simulink model "plant_block_swing_catch"  (R2013a)
settings: Solver=ode1  StartTime=0.0  StopTime=420  RelTol=1e-3
undefined symbols (not defined in the file or in its folder): magnitude
libraries: simulink x11
settings Model: SimulationMode=external  ExtModeTrigDuration=50000  Creator=Dro  LastModifiedBy=s4358046
settings DataIOCC: LimitDataPoints=off  SignalLoggingSaveFormat=ModelDataLogs  SignalLoggingName=sigsOut
settings OptimizationCC: ExpressionDepthLimit=2147483647  InitFltsAndDblsToZero=on
settings DebuggingCC: SaveWithParameterizedLinksMsg=none  SignalResolutionControl=TryResolveAllWithWarning  SolverPrmCheckMsg=none  MultiTaskDSMMsg=warning  MultiTaskCondExecSysMsg=none  FcnCallInpInsideContextMsg=UseLocalSettings  StrictBusMsg=None
settings RTWCC: SystemTargetFile=rtwin.tlc  TemplateMakefile=rtwin.tmf  Description=Real-Time Windows Target  ProcessScript=rtwin_make_rtw_hook  IncludeERTFirstTime=on
settings RTWinTargetCC: TargetFcnLib=ansi_tfl_tmw.mat  TargetLibSuffix=_rtwin.lib  TargetPreCompLibLocation=C:\Program Files\MATLAB\R2013a\toolbox\rtw\targets\rtwin\lib\win64  CodeReplacementLibrary=ANSI_C  ModelReferenceCompliant=off  CompOptLevelCompliant=off  RTWinDir=C:/PROGRA~1/MATLAB/R2013a/toolbox/rtw/targets/rtwin  TargetArch=win64

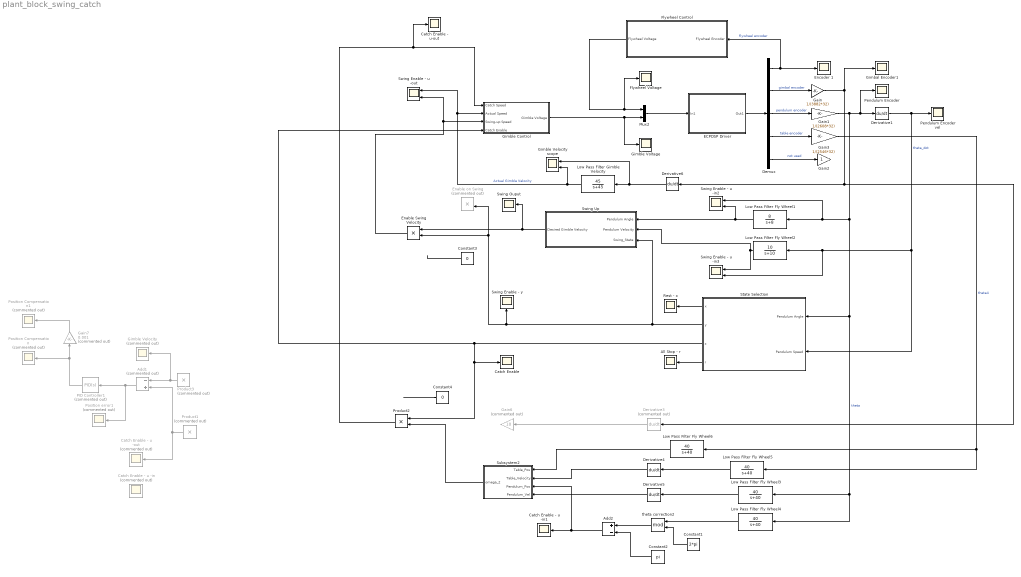
== system plant_block_swing_catch ==
  Add1 : Sum  Commented=on  Inputs=-+
  Add2 : Sum  Inputs=+-
  All Stop - r : Scope
      settings: YMin=-10  YMax=10  SaveName=ScopeData33
  Catch Enable : Scope
      settings: YMin=-10  YMax=10  SaveName=ScopeData12
  Catch Enable - u -in : Scope  Commented=on
      settings: YMin=-10  YMax=10  SaveName=ScopeData2
  Catch Enable - u -in1 : Scope
      settings: YMin=-10  YMax=10  SaveName=ScopeData26
  Catch Enable - u -out : Scope  Commented=on
      settings: YMin=-10  YMax=10  SaveName=ScopeData8
  Catch Enable - u-out : Scope
      settings: YMin=-10  YMax=10  SaveName=ScopeData20
  Constant1 : Constant  Value=2*pi
  Constant2 : Constant  Value=pi
  Constant3 : Constant  Value=0
  Constant4 : Constant  Value=0
  Demux : Demux  Outputs=5
  Derivative{1,4..6} (4 alike) : Derivative
  Derivative3 : Derivative  Commented=on
  ECPDSP Driver : Subsystem  mask{BaseAddr='0xC000', STime=0.008, TimeOutPer=500, HWAccess=on}
      mask prompts: BaseAddr "Base I/O Address"; STime "Sample Time (Sec)"; TimeOutPer "Timeout Period (500 ~ 2000)"; HWAccess "Hardware Access"
      mask Display: color('black');disp('ECPDSP Driver\n upto\n 4 Encs(ADC Channels)\n and 2 Dacs')
  Enable Swing Velocity : Product
  Enable on Swing : Product  Commented=on
  Encoder 1 : Scope
      settings: YMin=1.5e+06  YMax=8.5e+06  SaveName=ScopeData3
  Flywheel Control : Subsystem
  Flywheel Voltage : Scope
      settings: YMin=30400  YMax=33600  SaveName=ScopeData6
  Gain : Gain  Gain=1/(3882*32)
  Gain1 : Gain  Gain=1/(2608*32)
  Gain2 : Gain
  Gain3 : Gain  Gain=1/(2546*32)
  Gain6 : Gain  Commented=on  Gain=10
  Gain7 : Gain  Commented=on  Gain=0.001
  Gimbal Encoder1 : Scope
      settings: YMin=-0.25  YMax=3.25  SaveName=ScopeData9
  Gimble Control : Subsystem
  Gimble Velocity : Scope  Commented=on
      settings: YMin=-10  YMax=10  SaveName=ScopeData10
  Gimble Velocity scope : Scope  NumInputPorts=2
      settings: YMin=-10~-5  YMax=10~5  SaveName=ScopeData32
  Gimble Voltage : Scope
      settings: TimeRange=4.21022074346109  YMin=-27910.40741056809  YMax=13910.18606424908  SaveName=ScopeData23
  Low Pass Filter Fly Wheel1 : TransferFcn  Numerator=[8]  Denominator=[1 8]
  Low Pass Filter Fly Wheel2 : TransferFcn  Numerator=[10]  Denominator=[1 10]
  Low Pass Filter Fly Wheel{3..6} (4 alike) : TransferFcn  Numerator=[40]  Denominator=[1 40]
  Low Pass Filter Gimble Velocity : TransferFcn  Numerator=[45]  Denominator=[1 45]
  Mux2 : Mux  Inputs=2
  PID Controller1 : simulink/Continuous/PID Controller  Commented=on  Controller=PID  TimeDomain=Continuous-time  SampleTime=1  IntegratorMethod=Forward Euler  FilterMethod=Forward Euler  Form=Parallel  P=200  I=50  D=0  N=100  InitialConditionSource=internal  InitialConditionForIntegrator=0  InitialConditionForFilter=0  ExternalReset=none  LimitOutput=off  UpperSaturationLimit=inf  LowerSaturationLimit=-inf  LinearizeAsGain=on  AntiWindupMode=none  Kb=1  TrackingMode=off  Kt=1  PParamMin=[]  PParamMax=[]  IParamMin=[]  IParamMax=[]  DParamMin=[]  DParamMax=[]  NParamMin=[]  NParamMax=[]  KbParamMin=[]  KbParamMax=[]  KtParamMin=[]  KtParamMax=[]  POutMin=[]  POutMax=[]  IOutMin=[]  IOutMax=[]  DOutMin=[]  DOutMax=[]  NOutMin=[]  NOutMax=[]  KbOutMin=[]  KbOutMax=[]  KtOutMin=[]  KtOutMax=[]  IntegratorOutMin=[]  IntegratorOutMax=[]  FilterOutMin=[]  FilterOutMax=[]  SumOutMin=[]  SumOutMax=[]  SumI1OutMin=[]  SumI1OutMax=[]  SumI2OutMin=[]  SumI2OutMax=[]  SumI3OutMin=[]  SumI3OutMax=[]  SumDOutMin=[]  SumDOutMax=[]  SaturationOutMin=[]  SaturationOutMax=[]  IntegratorContinuousStateAttributes=''  IntegratorStateMustResolveToSignalObject=off  IntegratorRTWStateStorageClass=Auto  FilterContinuousStateAttributes=''  FilterStateMustResolveToSignalObject=off  FilterRTWStateStorageClass=Auto
  Pendulum Encoder : Scope
      settings: YMin=-3.175  YMax=-3.1  SaveName=ScopeData5
  Pendulum Encoder vel : Scope
      settings: YMin=-0.25  YMax=3.25  SaveName=ScopeData19
  Position Compensation : Scope  Commented=on
      settings: YMin=-10  YMax=10  SaveName=ScopeData11
  Position Compensation1 : Scope  Commented=on
      settings: YMin=-10  YMax=10  SaveName=ScopeData13
  Position error1 : Scope  Commented=on
      settings: YMin=-10  YMax=10  SaveName=ScopeData14
  Product1 : Product  Commented=on
  Product2 : Product
  Product3 : Product  Commented=on
  Rest - x : Scope
      settings: YMin=-10  YMax=10  SaveName=ScopeData15
  State Selection : Subsystem
  Subsystem2 : Subsystem
  Swing Enable - u -in2 : Scope  NumInputPorts=2
      settings: YMin=-10~-5  YMax=10~5  SaveName=ScopeData30
  Swing Enable - u -in3 : Scope  NumInputPorts=2
      settings: YMin=-10~-5  YMax=10~5  SaveName=ScopeData31
  Swing Enable - u -out : Scope  NumInputPorts=2
      settings: YMin=-10~-5  YMax=10~5  SaveName=ScopeData18
  Swing Enable - y : Scope
      settings: YMin=-10  YMax=10  SaveName=ScopeData16
  Swing Ouput : Scope
      settings: YMin=-10  YMax=10  SaveName=ScopeData17
  Swing Up : Subsystem
  theta correction2 : Math  Operator=mod  SaturateOnIntegerOverflow=on
  wires:
  ECPDSP Driver/1(Out1) -> Demux/1
  Demux/1 -> Encoder 1/1, Flywheel Control/1(Flywheel Encoder)  "flywheel encoder"
  Demux/2 -> Gain/1  "gimbal encoder"
  Demux/3 -> Gain1/1  "pendulum encoder"
  Demux/4 -> Gain3/1  "table encoder"
  Demux/5 -> Gain2/1  "not used"
  Derivative1/1 -> State Selection/2(Pendulum Speed), Swing Enable - u -in3/2, Low Pass Filter Fly Wheel2/1, Pendulum Encoder vel/1  "theta_dot"
  Gain1/1 -> Low Pass Filter Fly Wheel3/1, Low Pass Filter Fly Wheel4/1, State Selection/1(Pendulum Angle), Swing Enable - u -in2/1, Low Pass Filter Fly Wheel1/1, Pendulum Encoder/1, Derivative1/1  "theta"
  Swing Up/1(Desired Gimble Velocity) -> Swing Ouput/1, Enable Swing Velocity/1
  Subsystem2/1(omega_2) -> Product2/2
  Derivative3/1 -> Gain6/1
  theta correction2/1 -> Add2/1
  Add2/1 -> Subsystem2/3(Pendulum_Pos), Catch Enable - u -in1/1
  Mux2/1 -> ECPDSP Driver/1(In1)
  Derivative4/1 -> Subsystem2/2(Table_Velocity)
  Constant1/1 -> theta correction2/2
  Constant2/1 -> Add2/2
  Derivative6/1 -> Low Pass Filter Gimble Velocity/1, Gimble Velocity scope/1
  Low Pass Filter Fly Wheel2/1 -> Swing Up/2(Pendulum Velocity), Swing Enable - u -in3/1
  Low Pass Filter Gimble Velocity/1 -> Gimble Velocity scope/2, Swing Enable - u -out/1, Gimble Control/2(Actual Speed)  "Actual Gimble Velocity"
  Low Pass Filter Fly Wheel1/1 -> Swing Enable - u -in2/2, Swing Up/1(Pendulum Angle)
  Enable Swing Velocity/1 -> Swing Enable - u -out/2, Gimble Control/3(Swing-up Speed)
  Flywheel Control/1(Flywheel Voltage) -> Flywheel Voltage/1, Mux2/1
  Gimble Control/1(Gimble Voltage) -> Mux2/2, Gimble Voltage/1
  State Selection/2(y) -> Enable Swing Velocity/2, Enable on Swing/2, Swing Enable - y/1, Swing Up/3(Swing_State)
  State Selection/1(x) -> Rest - x/1
  State Selection/4(r) -> All Stop - r/1
  Gain3/1 -> Low Pass Filter Fly Wheel5/1, Low Pass Filter Fly Wheel6/1  "theta4"
  Constant3/1 -> ?
  Gain/1 -> Derivative3/1, Derivative6/1, Gimbal Encoder1/1
  ? -> Catch Enable - u -in/1
  ? -> Product1/2
  Add1/1 -> Position error1/1, PID Controller1/1
  Product3/1 -> Gimble Velocity/1, Add1/1
  Product1/1 -> Catch Enable - u -out/1, Add1/2
  ? -> Product3/1
  PID Controller1/1 -> Position Compensation/1, Gain7/1
  Gain7/1 -> Position Compensation1/1
  ? -> Product3/2
  ? -> Product1/1
  Product2/1 -> Catch Enable - u-out/1, Gimble Control/1(Catch Speed)
  Constant4/1 -> ?
  State Selection/3(z) -> Gimble Control/4(Catch Enable), Product2/1, Catch Enable/1
  Low Pass Filter Fly Wheel4/1 -> theta correction2/1
  Derivative5/1 -> Subsystem2/4(Pendulum_Vel)
  Low Pass Filter Fly Wheel3/1 -> Derivative5/1
  Low Pass Filter Fly Wheel5/1 -> Derivative4/1
  Low Pass Filter Fly Wheel6/1 -> Subsystem2/1(Table_Pos)

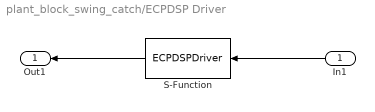
== system plant_block_swing_catch/ECPDSP Driver ==
  In1 : Inport
  S-Function : S-Function  FunctionName=ECPDSPDriver  Parameters=BaseAddr,STime,TimeOutPer,HWAccess  EnableBusSupport=off
  Out1 : Outport
  wires:
  In1/1 -> S-Function/1
  S-Function/1 -> Out1/1

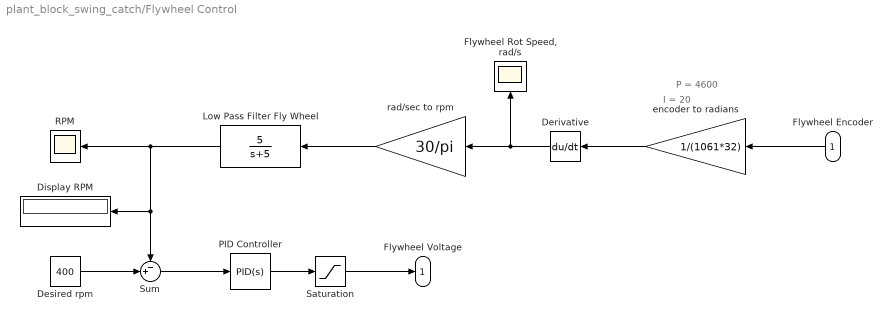
== system plant_block_swing_catch/Flywheel Control ==
  note: I = 20
  note: P = 4600
  Flywheel Encoder : Inport
  Derivative : Derivative
  Desired rpm : Constant  Value=400
  Display RPM : Display
  "Flywheel Rot Speed, rad/s" : Scope
      settings: SaveName=ScopeData4
  Low Pass Filter Fly Wheel : TransferFcn  Numerator=[5]  Denominator=[1 5]
  PID Controller : simulink/Continuous/PID Controller  Controller=PID  TimeDomain=Continuous-time  SampleTime=1  IntegratorMethod=Forward Euler  FilterMethod=Forward Euler  Form=Parallel  P=4600  I=20  D=0  N=100  InitialConditionSource=internal  InitialConditionForIntegrator=0  InitialConditionForFilter=0  ExternalReset=none  LimitOutput=off  UpperSaturationLimit=inf  LowerSaturationLimit=-inf  LinearizeAsGain=on  AntiWindupMode=none  Kb=1  TrackingMode=off  Kt=1  PParamMin=[]  PParamMax=[]  IParamMin=[]  IParamMax=[]  DParamMin=[]  DParamMax=[]  NParamMin=[]  NParamMax=[]  KbParamMin=[]  KbParamMax=[]  KtParamMin=[]  KtParamMax=[]  POutMin=[]  POutMax=[]  IOutMin=[]  IOutMax=[]  DOutMin=[]  DOutMax=[]  NOutMin=[]  NOutMax=[]  KbOutMin=[]  KbOutMax=[]  KtOutMin=[]  KtOutMax=[]  IntegratorOutMin=[]  IntegratorOutMax=[]  FilterOutMin=[]  FilterOutMax=[]  SumOutMin=[]  SumOutMax=[]  SumI1OutMin=[]  SumI1OutMax=[]  SumI2OutMin=[]  SumI2OutMax=[]  SumI3OutMin=[]  SumI3OutMax=[]  SumDOutMin=[]  SumDOutMax=[]  SaturationOutMin=[]  SaturationOutMax=[]  IntegratorContinuousStateAttributes=''  IntegratorStateMustResolveToSignalObject=off  IntegratorRTWStateStorageClass=Auto  FilterContinuousStateAttributes=''  FilterStateMustResolveToSignalObject=off  FilterRTWStateStorageClass=Auto
  RPM : Scope
      settings: YMin=401.6  YMax=403.9
  Saturation : Saturate  UpperLimit=32000  LowerLimit=-32000
  Sum : Sum  Inputs=-+|
  encoder to radians : Gain  Gain=1/(1061*32)
  rad/sec to rpm : Gain  Gain=30/pi
  Flywheel Voltage : Outport
  wires:
  Saturation/1 -> Flywheel Voltage/1
  Sum/1 -> PID Controller/1
  Desired rpm/1 -> Sum/2
  rad/sec to rpm/1 -> Low Pass Filter Fly Wheel/1
  Derivative/1 -> "Flywheel Rot Speed, rad/s"/1, rad/sec to rpm/1
  encoder to radians/1 -> Derivative/1
  Low Pass Filter Fly Wheel/1 -> Sum/1, Display RPM/1, RPM/1
  PID Controller/1 -> Saturation/1
  Flywheel Encoder/1 -> encoder to radians/1

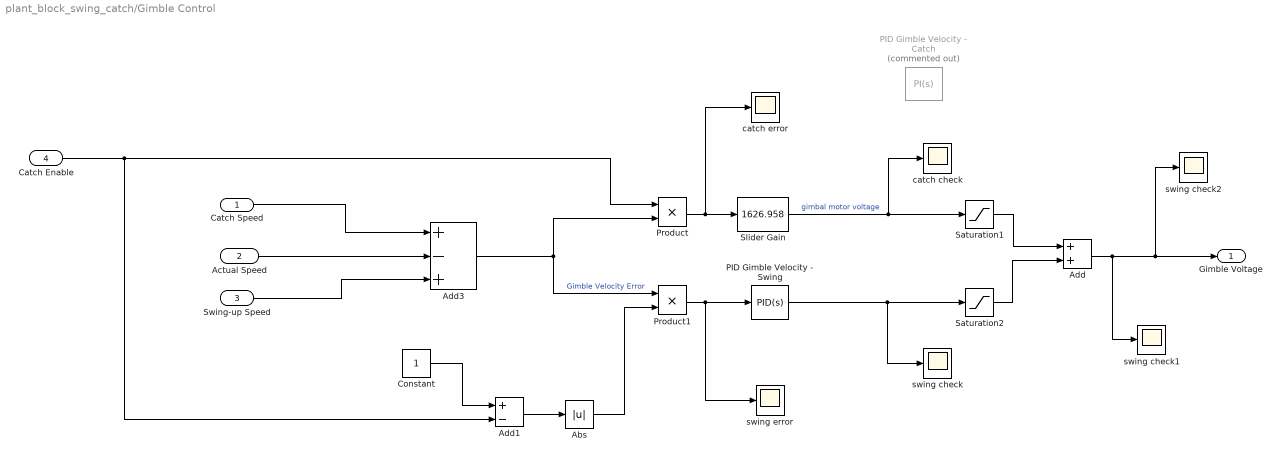
== system plant_block_swing_catch/Gimble Control ==
  Catch Speed : Inport
  Actual Speed : Inport  Port=2
  Swing-up Speed : Inport  Port=3
  Catch Enable : Inport  Port=4
  Abs : Abs
  Add : Sum
  Add1 : Sum  Inputs=+-
  Add3 : Sum  Inputs=+-+
  Constant : Constant
  PID Gimble Velocity - Catch : simulink/Continuous/PID Controller  Commented=on  Controller=PI  TimeDomain=Continuous-time  SampleTime=1  IntegratorMethod=Forward Euler  FilterMethod=Forward Euler  Form=Parallel  P=1000  I=0  D=0  N=100  InitialConditionSource=internal  InitialConditionForIntegrator=0  InitialConditionForFilter=0  ExternalReset=none  LimitOutput=off  UpperSaturationLimit=inf  LowerSaturationLimit=-inf  LinearizeAsGain=on  AntiWindupMode=none  Kb=1  TrackingMode=off  Kt=1  PParamMin=[]  PParamMax=[]  IParamMin=[]  IParamMax=[]  DParamMin=[]  DParamMax=[]  NParamMin=[]  NParamMax=[]  KbParamMin=[]  KbParamMax=[]  KtParamMin=[]  KtParamMax=[]  POutMin=[]  POutMax=[]  IOutMin=[]  IOutMax=[]  DOutMin=[]  DOutMax=[]  NOutMin=[]  NOutMax=[]  KbOutMin=[]  KbOutMax=[]  KtOutMin=[]  KtOutMax=[]  IntegratorOutMin=[]  IntegratorOutMax=[]  FilterOutMin=[]  FilterOutMax=[]  SumOutMin=[]  SumOutMax=[]  SumI1OutMin=[]  SumI1OutMax=[]  SumI2OutMin=[]  SumI2OutMax=[]  SumI3OutMin=[]  SumI3OutMax=[]  SumDOutMin=[]  SumDOutMax=[]  SaturationOutMin=[]  SaturationOutMax=[]  IntegratorContinuousStateAttributes=''  IntegratorStateMustResolveToSignalObject=off  IntegratorRTWStateStorageClass=Auto  FilterContinuousStateAttributes=''  FilterStateMustResolveToSignalObject=off  FilterRTWStateStorageClass=Auto
  PID Gimble Velocity - Swing : simulink/Continuous/PID Controller  Controller=PID  TimeDomain=Continuous-time  SampleTime=1  IntegratorMethod=Forward Euler  FilterMethod=Forward Euler  Form=Parallel  P=12000  I=2500  D=0  N=100  InitialConditionSource=internal  InitialConditionForIntegrator=0  InitialConditionForFilter=0  ExternalReset=none  LimitOutput=off  UpperSaturationLimit=inf  LowerSaturationLimit=-inf  LinearizeAsGain=on  AntiWindupMode=none  Kb=1  TrackingMode=off  Kt=1  PParamMin=[]  PParamMax=[]  IParamMin=[]  IParamMax=[]  DParamMin=[]  DParamMax=[]  NParamMin=[]  NParamMax=[]  KbParamMin=[]  KbParamMax=[]  KtParamMin=[]  KtParamMax=[]  POutMin=[]  POutMax=[]  IOutMin=[]  IOutMax=[]  DOutMin=[]  DOutMax=[]  NOutMin=[]  NOutMax=[]  KbOutMin=[]  KbOutMax=[]  KtOutMin=[]  KtOutMax=[]  IntegratorOutMin=[]  IntegratorOutMax=[]  FilterOutMin=[]  FilterOutMax=[]  SumOutMin=[]  SumOutMax=[]  SumI1OutMin=[]  SumI1OutMax=[]  SumI2OutMin=[]  SumI2OutMax=[]  SumI3OutMin=[]  SumI3OutMax=[]  SumDOutMin=[]  SumDOutMax=[]  SaturationOutMin=[]  SaturationOutMax=[]  IntegratorContinuousStateAttributes=''  IntegratorStateMustResolveToSignalObject=off  IntegratorRTWStateStorageClass=Auto  FilterContinuousStateAttributes=''  FilterStateMustResolveToSignalObject=off  FilterRTWStateStorageClass=Auto
  Product : Product
  Product1 : Product
  Saturation1 : Saturate  UpperLimit=40000  LowerLimit=-40000
  Saturation2 : Saturate  UpperLimit=9500  LowerLimit=-9500
  Slider Gain : simulink/Math Operations/Slider Gain  low=0  gain=1626.958  high=2000
  catch check : Scope
      settings: SaveName=ScopeData21
  catch error : Scope
      settings: SaveName=ScopeData24
  swing check : Scope
      settings: SaveName=ScopeData22
  swing check1 : Scope
      settings: SaveName=ScopeData27
  swing check2 : Scope
      settings: SaveName=ScopeData37
  swing error : Scope
      settings: SaveName=ScopeData25
  Gimble Voltage : Outport
  wires:
  Actual Speed/1 -> Add3/2
  Add3/1 -> Product1/1, Product/2  "Gimble Velocity Error"
  Slider Gain/1 -> Saturation1/1, catch check/1  "gimbal motor voltage"
  Add/1 -> swing check1/1, swing check2/1, Gimble Voltage/1
  PID Gimble Velocity - Swing/1 -> Saturation2/1, swing check/1
  Product/1 -> Slider Gain/1, catch error/1
  Catch Speed/1 -> Add3/1
  Constant/1 -> Add1/1
  Catch Enable/1 -> Add1/2, Product/1
  Add1/1 -> Abs/1
  Abs/1 -> Product1/2
  Product1/1 -> swing error/1, PID Gimble Velocity - Swing/1
  Swing-up Speed/1 -> Add3/3
  Saturation1/1 -> Add/1
  Saturation2/1 -> Add/2

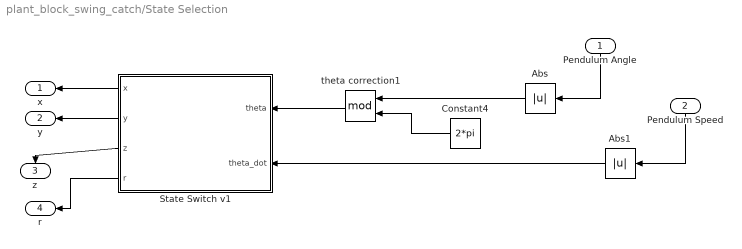
== system plant_block_swing_catch/State Selection ==
  Pendulum Angle : Inport
  Pendulum Speed : Inport  Port=2
  Abs : Abs
  Abs1 : Abs
  Constant4 : Constant  Value=2*pi
  State Switch v1 : Stateflow chart  TreatAsAtomicUnit=on
  theta correction1 : Math  Operator=mod  SaturateOnIntegerOverflow=on
  x : Outport
  y : Outport  Port=2
  z : Outport  Port=3
  r : Outport  Port=4
  wires:
  Pendulum Angle/1 -> Abs/1
  Pendulum Speed/1 -> Abs1/1
  Abs1/1 -> State Switch v1/2(theta_dot)
  State Switch v1/2(y) -> y/1
  State Switch v1/4(r) -> r/1
  State Switch v1/1(x) -> x/1
  theta correction1/1 -> State Switch v1/1(theta)
  Constant4/1 -> theta correction1/2
  Abs/1 -> theta correction1/1
  State Switch v1/3(z) -> z/1

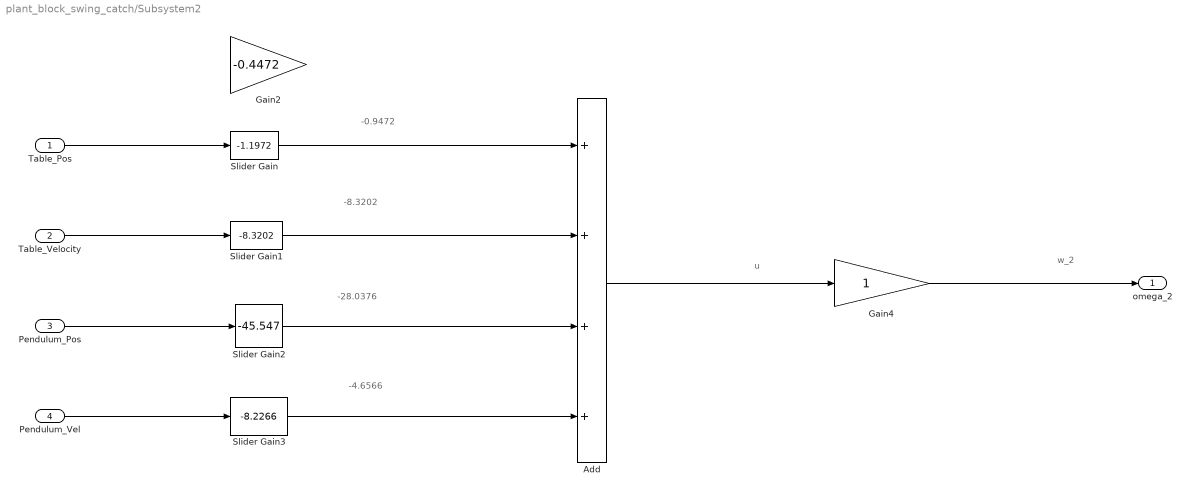
== system plant_block_swing_catch/Subsystem2 ==
  note: -4.6566
  note: -28.0376
  note: -8.3202
  note: -0.9472
  note: w_2
  note: u
  Table_Pos : Inport
  Table_Velocity : Inport  Port=2
  Pendulum_Pos : Inport  Port=3
  Pendulum_Vel : Inport  Port=4
  Add : Sum  Inputs=++++
  Gain2 : Gain  Gain=-0.4472
  Gain4 : Gain
  Slider Gain : simulink/Math Operations/Slider Gain  low=-20  gain=-1.1972  high=5
  Slider Gain1 : simulink/Math Operations/Slider Gain  low=-30  gain=-8.3202  high=1
  Slider Gain2 : simulink/Math Operations/Slider Gain  low=-80  gain=-45.547  high=1
  Slider Gain3 : simulink/Math Operations/Slider Gain  low=-20  gain=-8.2266  high=1
  omega_2 : Outport
  wires:
  Slider Gain/1 -> Add/1
  Slider Gain1/1 -> Add/2
  Table_Pos/1 -> Slider Gain/1
  Table_Velocity/1 -> Slider Gain1/1
  Slider Gain2/1 -> Add/3
  Slider Gain3/1 -> Add/4
  Pendulum_Pos/1 -> Slider Gain2/1
  Pendulum_Vel/1 -> Slider Gain3/1
  Add/1 -> Gain4/1
  Gain4/1 -> omega_2/1

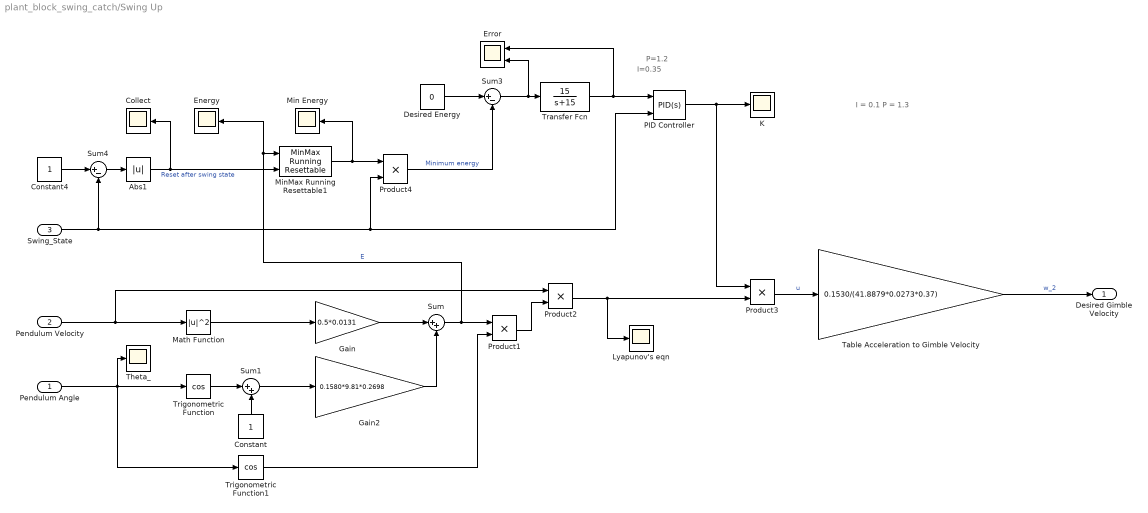
== system plant_block_swing_catch/Swing Up ==
  note: I=0.35
  note: P=1.2
  note: I = 0.1
      | P = 1.3
  Pendulum Angle : Inport
  Pendulum Velocity : Inport  Port=2
  Swing_State : Inport  Port=3
  Abs1 : Abs
  Collect : Scope
      settings: YMin=0.82  YMax=0.8575  SaveName=ScopeData35
  Constant : Constant
  Constant4 : Constant
  Desired Energy : Constant  Value=0
  Energy : Scope
      settings: YMin=0.82  YMax=0.8575  SaveName=ScopeData7
  Error : Scope  NumInputPorts=2
      settings: YMin=0.82~-5  YMax=0.8575~5  SaveName=ScopeData36
  Gain : Gain  Gain=0.5*0.0131
  Gain2 : Gain  Gain=0.1580*9.81*0.2698
  K : Scope
      settings: YMin=-0.00209088  YMax=-0.00209088  SaveName=ScopeData29
  Lyapunov's eqn : Scope
      settings: YMin=-10  YMax=10
  Math Function : Math  Operator=magnitude^2  SaturateOnIntegerOverflow=on
  Min Energy : Scope
      settings: YMin=0.82  YMax=0.8575  SaveName=ScopeData34
  MinMax Running Resettable1 : simulink/Math Operations/MinMax Running Resettable  Function=min  vinit=0.85
  PID Controller : simulink/Continuous/PID Controller  Controller=PID  TimeDomain=Continuous-time  SampleTime=1  IntegratorMethod=Forward Euler  FilterMethod=Forward Euler  Form=Parallel  P=0.5  I=0.15  D=0  N=100  InitialConditionSource=internal  InitialConditionForIntegrator=0  InitialConditionForFilter=0  ExternalReset=falling  LimitOutput=off  UpperSaturationLimit=inf  LowerSaturationLimit=-inf  LinearizeAsGain=on  AntiWindupMode=none  Kb=1  TrackingMode=off  Kt=1  PParamMin=[]  PParamMax=[]  IParamMin=[]  IParamMax=[]  DParamMin=[]  DParamMax=[]  NParamMin=[]  NParamMax=[]  KbParamMin=[]  KbParamMax=[]  KtParamMin=[]  KtParamMax=[]  POutMin=[]  POutMax=[]  IOutMin=[]  IOutMax=[]  DOutMin=[]  DOutMax=[]  NOutMin=[]  NOutMax=[]  KbOutMin=[]  KbOutMax=[]  KtOutMin=[]  KtOutMax=[]  IntegratorOutMin=[]  IntegratorOutMax=[]  FilterOutMin=[]  FilterOutMax=[]  SumOutMin=[]  SumOutMax=[]  SumI1OutMin=[]  SumI1OutMax=[]  SumI2OutMin=[]  SumI2OutMax=[]  SumI3OutMin=[]  SumI3OutMax=[]  SumDOutMin=[]  SumDOutMax=[]  SaturationOutMin=[]  SaturationOutMax=[]  IntegratorContinuousStateAttributes=''  IntegratorStateMustResolveToSignalObject=off  IntegratorRTWStateStorageClass=Auto  FilterContinuousStateAttributes=''  FilterStateMustResolveToSignalObject=off  FilterRTWStateStorageClass=Auto
  Product{1..4} (4 alike) : Product
  Sum : Sum  Inputs=|++
  Sum1 : Sum  Inputs=|++
  Sum3 : Sum  Inputs=|+-
  Sum4 : Sum  Inputs=|+-
  Table Acceleration to Gimble Velocity : Gain  Gain=0.1530/(41.8879*0.0273*0.37)
  Theta_ : Scope
      settings: YMin=-10  YMax=10  SaveName=ScopeData28
  Transfer Fcn : TransferFcn  Numerator=[15]  Denominator=[1 15]
  Trigonometric Function : Trigonometry  Operator=cos
  Trigonometric Function1 : Trigonometry  Operator=cos
  Desired Gimble Velocity : Outport
  wires:
  Pendulum Velocity/1 -> Math Function/1, Product2/1
  Math Function/1 -> Gain/1
  Gain/1 -> Sum/1
  Product3/1 -> Table Acceleration to Gimble Velocity/1  "u"
  Trigonometric Function/1 -> Sum1/1
  Constant/1 -> Sum1/2
  Sum1/1 -> Gain2/1
  Sum/1 -> Product1/1, Energy/1, MinMax Running Resettable1/1  "E"
  Trigonometric Function1/1 -> Product1/2
  Product1/1 -> Product2/2
  Gain2/1 -> Sum/2
  Product2/1 -> Product3/2, Lyapunov's eqn/1
  Table Acceleration to Gimble Velocity/1 -> Desired Gimble Velocity/1  "w_2"
  Pendulum Angle/1 -> Theta_/1, Trigonometric Function1/1, Trigonometric Function/1
  Sum3/1 -> Error/2, Transfer Fcn/1
  Desired Energy/1 -> Sum3/1
  Product4/1 -> Sum3/2  "Minimum energy"
  Swing_State/1 -> PID Controller/2, Product4/2, Sum4/2
  Constant4/1 -> Sum4/1
  Sum4/1 -> Abs1/1
  MinMax Running Resettable1/1 -> Product4/1, Min Energy/1
  PID Controller/1 -> Product3/1, K/1
  Transfer Fcn/1 -> Error/1, PID Controller/1
  Abs1/1 -> Collect/1, MinMax Running Resettable1/2  "Reset after swing state"

== stateflow chart plant_block_swing_catch/State Selection/State Switch v1 ==
  state Swing
    entry:
    x = 0,
    y = 1,
    z = 0,
    r = 0;
  state Rest
    entry:
    x = 1,
    y = 0,
    z = 0;
    r = 0;
  state Catch
    entry:
    x = 0,
    y = 0,
    z = 1;
    r = 0;
  state ReSwing
    entry:
    x = 1,
    y = 0,
    z = 0;
    r = 1;
  (default) -> Rest
  Rest -> Swing : [theta > 0.12 & theta_dot > 0.12]
  ReSwing -> Swing : [theta_dot < 2 & (theta < (pi/4) | theta > (2*pi- pi/4))]
  Swing -> Rest [order 2] : [theta < 0.12 & theta_dot < 0.12]
  Swing -> Catch [order 1] : [(3.14 - (3.14/10)) < theta & theta < (3.14 + (3.14/10))]
  Catch -> ReSwing [order 1] : [theta_dot > 8 & theta > (pi-pi/8) & theta < (pi+pi/8)]
  Catch -> ReSwing [order 2] : [theta < (3.14 - (3.14/10)) | theta > (3.14 + (3.14/10))]
  data: x output; y output; z output; theta input; theta_dot input; r output
